simulink model "prova_P2_velocidade"  (R2020a)
settings: Solver=VariableStepAuto  StartTime=0.0  StopTime=50.0  MaxStep=1e-3  RelTol=1e-3
values from neighbouring files (symbols this model uses):
  Tz = 0.001    [ResultadosFinais.mat]
settings Model: Creator=jguil  LastModifiedBy=jguil

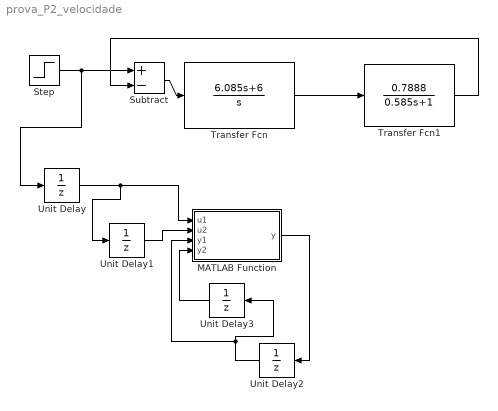
== system prova_P2_velocidade ==
  MATLAB Function : MATLAB Function  TreatAsAtomicUnit=on
  Step : Step  SampleTime=0
  Subtract : Sum  Inputs=+-
  Transfer Fcn : TransferFcn  Numerator=[6.085 6]  Denominator=[1 0]
  Transfer Fcn1 : TransferFcn  Numerator=0.7888  Denominator=[0.585 1]
  Unit Delay{,1..3} (4 alike) : UnitDelay  SampleTime=Tz  HasFrameUpgradeWarning=on
  wires:
  Subtract/1 -> Transfer Fcn/1
  Transfer Fcn/1 -> Transfer Fcn1/1
  Transfer Fcn1/1 -> Subtract/2
  Step/1 -> Unit Delay/1, Subtract/1
  Unit Delay2/1 -> MATLAB Function/3(y1), Unit Delay3/1
  MATLAB Function/1(y) -> Unit Delay2/1
  Unit Delay3/1 -> MATLAB Function/4(y2)
  Unit Delay/1 -> Unit Delay1/1, MATLAB Function/1(u1)
  Unit Delay1/1 -> MATLAB Function/2(u2)

== matlab function prova_P2_velocidade/MATLAB Function ==
  data: u1 input; y output; u2 input; y1 input; y2 input
function y = aprox(u1,u2,y1,y2)

y = 1.9900944048*y1 -0.9901024885*y2 +0.00819765369*u1-0.00818956998*u2;
